simulink model "Cryogenic_ORC"  (R2017a)
settings: Solver=VariableStepAuto  StartTime=0.0  StopTime=10.0  RelTol=1e-3
libraries: simCryogenics_lib x15, nesl_utility x5, fl_lib x3
settings Model: Creator=romain  LastModifiedBy=romain

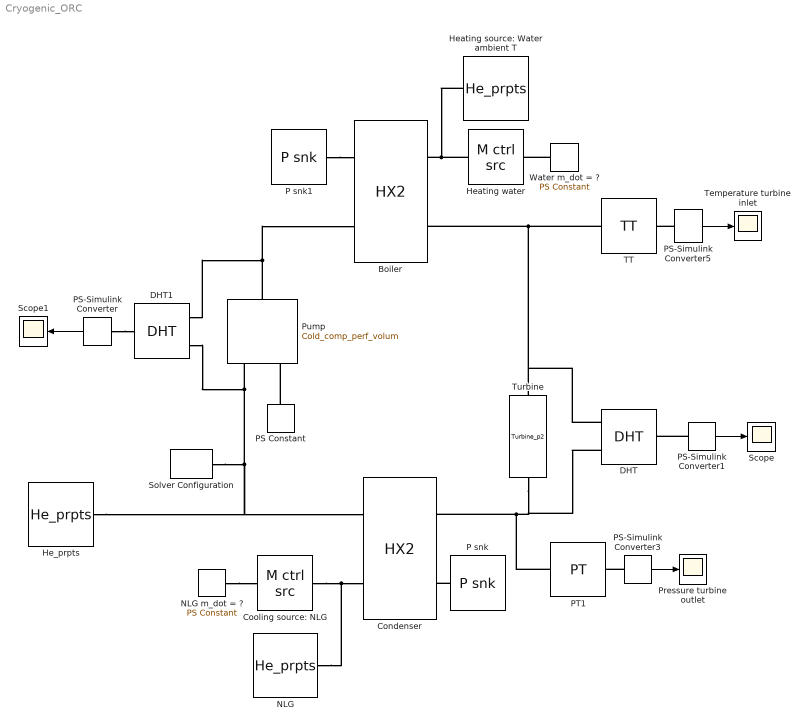
== system Cryogenic_ORC ==
  Boiler : simCryogenics_lib/Elements/HX2  N=6  Vh=2.3e-3 m^3  Vc=2.3e-3 m^3  M=13 kg  Kh=0.6 s*bar/kg  Kc=0.35 s*bar/kg  h=480 J/s/K  Th0=10 K  Ph0=16 bar  Mh0=0.037 kg/s  Tc0=4.5 K  Pc0=1.1 bar  Mc0=0.037 kg/s
  Condenser : simCryogenics_lib/Elements/HX2  N=6  Vh=2.3e-3 m^3  Vc=2.3e-3 m^3  M=13 kg  Kh=0.6 s*bar/kg  Kc=0.35 s*bar/kg  h=480 J/s/K  Th0=10 K  Ph0=16 bar  Mh0=0.037 kg/s  Tc0=4.5 K  Pc0=1.1 bar  Mc0=0.037 kg/s
  Cooling source: NLG : simCryogenics_lib/Sources_Sinks/M ctrl src
  DHT : simCryogenics_lib/Sensors/DHT
  DHT1 : simCryogenics_lib/Sensors/DHT
  He_prpts : simCryogenics_lib/Utilities/He_prpts  P_min=0.01 bar  P_max=50 bar  T_min=1 K  T_max=350 K  N=100
  Heating source: Water ambient T : simCryogenics_lib/Utilities/He_prpts  P_min=0.01 bar  P_max=50 bar  T_min=1 K  T_max=350 K  N=100
  Heating water : simCryogenics_lib/Sources_Sinks/M ctrl src
  NLG : simCryogenics_lib/Utilities/He_prpts  P_min=0.01 bar  P_max=50 bar  T_min=1 K  T_max=350 K  N=100
  NLG m_dot = ? : fl_lib/Physical Signals/Sources/PS Constant  constant=0.03
  P snk : simCryogenics_lib/Sources_Sinks/P snk  P=0 bar
  P snk1 : simCryogenics_lib/Sources_Sinks/P snk  P=0 bar
  PS Constant : fl_lib/Physical Signals/Sources/PS Constant  constant=0.03
  PS-Simulink Converter{,1,3,5} (4 alike) : nesl_utility/PS-Simulink Converter  PhysicalDomain=network_engine_domain  SubClassName=ps_output  LeftPortType=input  RightPortType=output  PseudoPeriodic=off  Frequencies=[]  Unit=1  AffineConversion=off
  PT1 : simCryogenics_lib/Sensors/PT
  Pressure turbine outlet : Scope
  Pump : simCryogenics_lib/Elements/Cold_comp_perf_volum  rho0=0 kg/m^3  eta=0.5  vol=0  Sin_specify=off  Sin_priority=None  Sin=0 kJ/kg  Sin_nominal_specify=off  Sin_nominal_unit=kJ/kg  Sin_nominal_value=1  HoutIs_specify=off  HoutIs_priority=None  HoutIs=0 kJ/kg  HoutIs_nominal_specify=off  HoutIs_nominal_unit=kJ/kg  HoutIs_nominal_value=1  rho_specify=off  rho_priority=None  rho=1 kg/m^3  rho_nominal_specify=off  rho_nominal_unit=kg/m^3  rho_nominal_value=1
  Scope : Scope
  Scope1 : Scope
  Solver Configuration : nesl_utility/Solver Configuration  PhysicalDomain=network_engine_domain  SubClassName=solver  LeftPortType=input  RightPortType=generic  Accelerate=off  Tones=[]  Harmonics=[]  SimulateNoise=off  Profile=off  UseLocalSampling=off  EnableSwitchedLinearOptims=on  FrequencyDomain=off  UseCCode=off  RelTol=0.001  AbsTol=1e-06  MinStep=1e-09  ToWorkspace=off  RevertToSquareIcSolve=off  NumHomotopyIterations=100  PhasorMode=off  PhasorModeNumHarmonics=1  OverrideAbsTol=off  DoDC=off  ResidualTolerance=1e-09  UseLocalSolver=off  LocalSolverChoice=NE_BACKWARD_EULER_ADVANCER  LocalSolverSampleTime=0.001  DoFixedCost=off  MaxNonlinIter=3  MaxModeIter=2  LinearAlgebra=Sparse  DelaysMemoryBudget=1024  AutomaticFiltering=on  FilteringTimeConstant=0.001
  TT : simCryogenics_lib/Sensors/TT  H_specify=off  H_priority=None  H=1 J/kg  H_nominal_specify=off  H_nominal_unit=J/kg  H_nominal_value=1
  Temperature turbine inlet : Scope
  Turbine : simCryogenics_lib/Elements/Turbine_p2  A=5e-5 m^2  D=0.0255 m  Mass=0.02 kg  cst_eff=0  eta0=0.8  Tin0=20 K  Pin0=16 bar  Pout0=1.2 bar  Ninit=2250 1/s  Nm=2250 rad/s  Q0=0 W  v0=0  I=0 kg*m^2  gamma_specify=off  gamma_priority=None  gamma=0  gamma_nominal_specify=off  gamma_nominal_unit=1  gamma_nominal_value=1  C_specify=off  C_priority=None  C=0  C_nominal_specify=off  C_nominal_unit=1  C_nominal_value=1  C_sq_specify=off  C_sq_priority=None  C_sq=0  C_sq_nominal_specify=off  C_sq_nominal_unit=1  C_sq_nominal_value=1  Z_specify=off  Z_priority=None  Z=0  Z_nominal_specify=off  Z_nominal_unit=1  Z_nominal_value=1  Cp_specify=off  Cp_priority=None  Cp=0 kJ/kg/K  Cp_nominal_specify=off  Cp_nominal_unit=kJ/kg/K  Cp_nominal_value=1  Sin_specify=off  Sin_priority=None  Sin=0 kJ/kg  Sin_nominal_specify=off  Sin_nominal_unit=kJ/kg  Sin_nominal_value=1  T_specify=off  T_priority=None  T=0 K  T_nominal_specify=off  T_nominal_unit=K  T_nominal_value=1  HoutIs_specify=off  HoutIs_priority=None  HoutIs=0 kJ/kg  HoutIs_nominal_specify=off  HoutIs_nominal_unit=kJ/kg  HoutIs_nominal_value=1  u1_specify=off  u1_priority=None  u1=0 m/s  u1_nominal_specify=off  u1_nominal_unit=m/s  u1_nominal_value=1  c1_specify=off  c1_priority=None  c1=0 m/s  c1_nominal_specify=off  c1_nominal_unit=m/s  c1_nominal_value=1  v_specify=off  v_priority=None  v=0  v_nominal_specify=off  v_nominal_unit=1  v_nominal_value=1  eta_specify=off  eta_priority=None  eta=0  eta_nominal_specify=off  eta_nominal_unit=1  eta_nominal_value=1  eta_var_specify=off  eta_var_priority=None  eta_var=0  eta_var_nominal_specify=off  eta_var_nominal_unit=1  eta_var_nominal_value=1  N_specify=off  N_priority=None  N=0 rad/s  N_nominal_specify=off  N_nominal_unit=rad/s  N_nominal_value=1  Q_specify=off  Q_priority=None  Q=0 W  Q_nominal_specify=off  Q_nominal_unit=W  Q_nominal_value=1  rp_crit_specify=off  rp_crit_priority=None  rp_crit=1  rp_crit_nominal_specify=off  rp_crit_nominal_unit=1  rp_crit_nominal_value=1  rp_c_specify=off  rp_c_priority=None  rp_c=1  rp_c_nominal_specify=off  rp_c_nominal_unit=1  rp_c_nominal_value=1  DHis_specify=off  DHis_priority=None  DHis=1 kJ/kg  DHis_nominal_specify=off  DHis_nominal_unit=kJ/kg  DHis_nominal_value=1
  Water m_dot = ? : fl_lib/Physical Signals/Sources/PS Constant  constant=0.03
  wires:
  PS-Simulink Converter5/1 -> Temperature turbine inlet/1
  PS-Simulink Converter1/1 -> Scope/1
  PS-Simulink Converter/1 -> Scope1/1
  PS-Simulink Converter3/1 -> Pressure turbine outlet/1
  connections:
  PT1/LConn1 -- DHT/LConn2 -- Turbine/RConn1 -- Condenser/LConn2
  Pump/RConn1 -- DHT1/LConn2 -- Boiler/LConn2
  TT/LConn1 -- DHT/LConn1 -- Turbine/LConn1 -- Boiler/RConn2
  DHT1/LConn1 -- He_prpts/RConn1 -- Condenser/RConn2 -- Solver Configuration/RConn1 -- Pump/LConn1
  PS-Simulink Converter1/LConn1 -- DHT/RConn1
  PS-Simulink Converter5/LConn1 -- TT/RConn1
  PS Constant/RConn1 -- Pump/LConn2
  PS-Simulink Converter/LConn1 -- DHT1/RConn1
  PS-Simulink Converter3/LConn1 -- PT1/RConn1
  Cooling source: NLG/RConn1 -- NLG/RConn1 -- Condenser/RConn1
  NLG m_dot = ?/RConn1 -- Cooling source: NLG/LConn1
  Heating water/RConn1 -- Heating source: Water ambient T/RConn1 -- Boiler/RConn1
  P snk/RConn1 -- Condenser/LConn1
  P snk1/RConn1 -- Boiler/LConn1
  Water m_dot = ?/RConn1 -- Heating water/LConn1
